simulink model "Fuzzy_pid_logic"  (R2025b)
settings: Solver=ode45  StartTime=0.0  StopTime=20  RelTol=1e-3
values from neighbouring files (symbols this model uses):
  ACE_norm = 0.20    (= 0.2)    [fuzzy_params.m]
  alpha = 0.002    [fuzzy_params.m]
  B = 0.425    [fuzzy_params.m]
  dACE_norm = 0.1    [fuzzy_params.m]
  Kd1 = Kp1 * Td1    (= 1.1799375)    [fuzzy_params.m]
  Kd2 = Kp2 * Td2    (= 0.2359875)    [fuzzy_params.m]
  Ki1 = Kp1 / Ti1    (= 0.00476720165263)    [fuzzy_params.m]
  Ki2 = Kp2 / Ti2    (= 0.000953440330526)    [fuzzy_params.m]
  Kp1 = 0.6 * Ku1    (= 0.15)    [fuzzy_params.m]
  Kp2 = 0.6 * Ku2    (= 0.03)    [fuzzy_params.m]
  Kps = 120    [fuzzy_params.m]
  Tg = 0.08    [fuzzy_params.m]
  TieGain = 2*pi*T12    (= 0.544123847602)    [fuzzy_params.m]
  Tps = 20    [fuzzy_params.m]
  Tt = 0.30    (= 0.3)    [fuzzy_params.m]
libraries: slpidlib x2, fuzblock x1
settings Model: Creator=parth  LastModifiedBy=parth
settings SolverCC: ZeroCrossAlgorithm=Adaptive
settings DebuggingCC: IgnoredZcDiagnostic=none

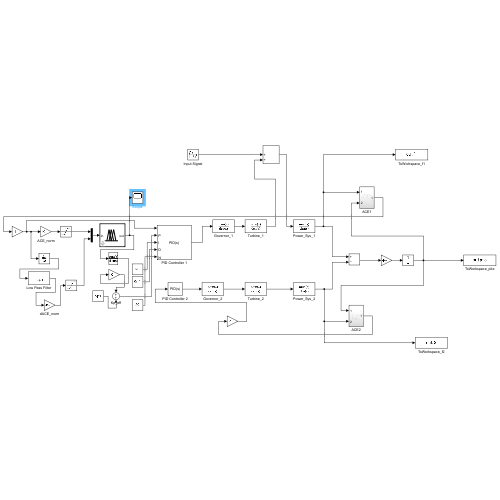
[thumbnail: Simulink's stored preview of the top-level diagram]
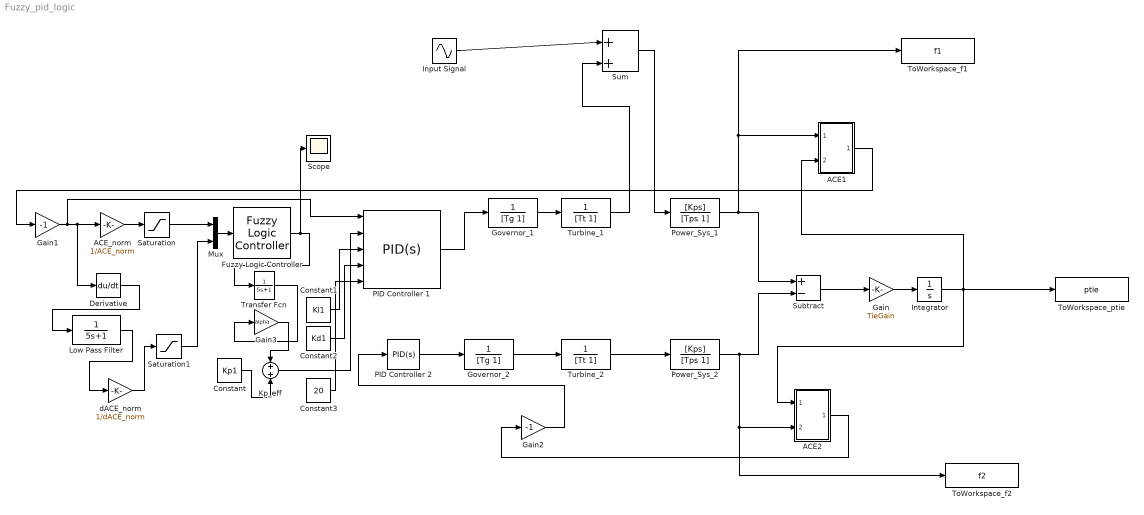
== system Fuzzy_pid_logic ==
  ACE1 : Subsystem
  ACE2 : Subsystem
  ACE_norm : Gain  Gain=1/ACE_norm
  Constant : Constant  Value=Kp1
  Constant1 : Constant  Value=Ki1
  Constant2 : Constant  Value=Kd1
  Constant3 : Constant  Value=20
  Derivative : Derivative  CoefficientInTFapproximation=1
  Fuzzy Logic Controller : fuzblock/Fuzzy Logic  Controller  FIS=fuzzy_pid  OutputSampleNumber=101  DataType=double  UseLookupTable=off  NumBreakpoints=10  FuzzifiedInputs=off  RuleFiringStrengths=off  RuleOutputs=off  AggregatedOutputs=off  SimulateUsing=Interpreted execution  OutOfRangeInputValueMessage=warning  NoRuleFiredMessage=warning  EmptyOutputFuzzySetMessage=warning
  Gain : Gain  Gain=TieGain
  Gain1 : Gain  Gain=-1
  Gain2 : Gain  Gain=-1
  Gain3 : Gain  Gain=alpha
  Governor_1 : TransferFcn  Denominator=[Tg 1]
  Governor_2 : TransferFcn  Denominator=[Tg 1]
  Input Signal : Sin  Amplitude=0.01  SampleTime=0
  Integrator : Integrator
  Kp_eff : Sum
  Low Pass Filter : TransferFcn  Denominator=[5 1]
  Mux : Mux  Inputs=2
  PID Controller 1 : slpidlib/PID Controller  Controller=PID  Form=Parallel  TimeDomain=Continuous-time  UseExternalTs=off  SampleTime=-1  IntegratorMethod=Forward Euler  FilterMethod=Forward Euler  ControllerParametersSource=external  P=Kp1  I=Ki1  UseKiTs=off  D=Kd1  UseExternalDerivativeSource=off  N=100  UseFilter=on  TunerSelectOption=Frequency Response Based  InitialConditionSource=internal  InitialConditionForIntegrator=0  InitialConditionForFilter=0  DifferentiatorICPrevScaledInput=0  ExternalReset=none  TrackingMode=off  Kt=1  LimitOutput=off  SatLimitsSource=internal  UpperSaturationLimit=inf  LowerSaturationLimit=-inf  LinearizeAsGain=on  AntiWindupMode=none  Kb=1  LimitIntegrator=off  UpperIntegratorSaturationLimit=inf  LowerIntegratorSaturationLimit=-inf  POutMin=[]  POutMax=[]  IOutMin=[]  IOutMax=[]  DOutMin=[]  DOutMax=[]  NOutMin=[]  NOutMax=[]  SumOutMin=[]  SumOutMax=[]  SaturationOutMin=[]  SaturationOutMax=[]  PParamMin=[]  PParamMax=[]  IParamMin=[]  IParamMax=[]  DParamMin=[]  DParamMax=[]  NParamMin=[]  NParamMax=[]  KbParamMin=[]  KbParamMax=[]  KtParamMin=[]  KtParamMax=[]  KbOutMin=[]  KbOutMax=[]  KtOutMin=[]  KtOutMax=[]  IntegratorOutMin=[]  IntegratorOutMax=[]  FilterOutMin=[]  FilterOutMax=[]  SumI1OutMin=[]  SumI1OutMax=[]  SumI2OutMin=[]  SumI2OutMax=[]  SumI3OutMin=[]  SumI3OutMax=[]  SumI4OutMin=[]  SumI4OutMax=[]  SumDOutMin=[]  SumDOutMax=[]  DifferentiatorOutMin=[]  DifferentiatorOutMax=[]  FilterDiffOutCoefMin=[]  FilterDiffOutCoefMax=[]  ReciprocalOutMin=[]  ReciprocalOutMax=[]  SumDenOutMin=[]  SumDenOutMax=[]  SumNumOutMin=[]  SumNumOutMax=[]  DivideOutMin=[]  DivideOutMax=[]  UdiffTsProdOutMin=[]  UdiffTsProdOutMax=[]  NTsProdOutMin=[]  NTsProdOutMax=[]  UintegralTsProdOutMin=[]  UintegralTsProdOutMax=[]  UngainTsProdOutMin=[]  UngainTsProdOutMax=[]  ClampingZeroOutDataTypeStr=Inherit: Inherit via back propagation  ClampingZeroOutMin=[]  ClampingZeroOutMax=[]  FilterDenConstantOutDataTypeStr=Inherit: Inherit via back propagation  FilterDenConstantOutMin=[]  FilterDenConstantOutMax=[]  PCopyOutDataTypeStr=Inherit: Inherit via back propagation  PCopyOutMin=[]  PCopyOutMax=[]  NCopyOutDataTypeStr=Inherit: Inherit via back propagation  NCopyOutMin=[]  NCopyOutMax=[]  IntegratorContinuousStateAttributes=''  IntegratorStateMustResolveToSignalObject=off  IntegratorRTWStateStorageClass=Auto  FilterContinuousStateAttributes=''  FilterStateMustResolveToSignalObject=off  FilterRTWStateStorageClass=Auto  ParallelPVariant=ExternalParameters  IdealPVariant=Disabled  IVariant=ExternalParameters  DVariant=ExternalParameters  IntegratorVariant=Continuous  SatVariant=Disabled  AWVariant=Passthrough  PCopyVariant=Disabled  TRVariant=Disabled  FdbkBlocksVariant=Forward  IdealPFdbkVariant=Disabled  SatFdbkVariant=Disabled  DerivativeFilterVariant=ContFilter  NVariant=ExternalParameters  NCopyVariant=Disabled  FilterICVariant=InternalICsFilter  IntegratorICVariant=InternalICs  ExternalResetVariant=Disabled  TRSumVariant=Passthrough  SumFdbkVariant=Disabled  SumVariant=Sum_PID  TsampFilterVariant=InternalTs  TsampNgainVariant=Passthrough  TsampIntegralVariant=Disabled_SignalSpec  ExternalSaturationOutDataTypeStr=Inherit: Same as second input  DerivativeSourceVariant=ErrorSignal  PreIntVariant=InternalPreInt
  PID Controller 2 : slpidlib/PID Controller  Controller=PID  Form=Parallel  TimeDomain=Continuous-time  UseExternalTs=off  SampleTime=-1  IntegratorMethod=Forward Euler  FilterMethod=Forward Euler  ControllerParametersSource=internal  P=Kp2  I=Ki2  UseKiTs=off  D=Kd2  UseExternalDerivativeSource=off  N=100  UseFilter=on  TunerSelectOption=Frequency Response Based  InitialConditionSource=internal  InitialConditionForIntegrator=0  InitialConditionForFilter=0  DifferentiatorICPrevScaledInput=0  ExternalReset=none  TrackingMode=off  Kt=1  LimitOutput=off  SatLimitsSource=internal  UpperSaturationLimit=inf  LowerSaturationLimit=-inf  LinearizeAsGain=on  AntiWindupMode=none  Kb=1  LimitIntegrator=off  UpperIntegratorSaturationLimit=inf  LowerIntegratorSaturationLimit=-inf  POutMin=[]  POutMax=[]  IOutMin=[]  IOutMax=[]  DOutMin=[]  DOutMax=[]  NOutMin=[]  NOutMax=[]  SumOutMin=[]  SumOutMax=[]  SaturationOutMin=[]  SaturationOutMax=[]  PParamMin=[]  PParamMax=[]  IParamMin=[]  IParamMax=[]  DParamMin=[]  DParamMax=[]  NParamMin=[]  NParamMax=[]  KbParamMin=[]  KbParamMax=[]  KtParamMin=[]  KtParamMax=[]  KbOutMin=[]  KbOutMax=[]  KtOutMin=[]  KtOutMax=[]  IntegratorOutMin=[]  IntegratorOutMax=[]  FilterOutMin=[]  FilterOutMax=[]  SumI1OutMin=[]  SumI1OutMax=[]  SumI2OutMin=[]  SumI2OutMax=[]  SumI3OutMin=[]  SumI3OutMax=[]  SumI4OutMin=[]  SumI4OutMax=[]  SumDOutMin=[]  SumDOutMax=[]  DifferentiatorOutMin=[]  DifferentiatorOutMax=[]  FilterDiffOutCoefMin=[]  FilterDiffOutCoefMax=[]  ReciprocalOutMin=[]  ReciprocalOutMax=[]  SumDenOutMin=[]  SumDenOutMax=[]  SumNumOutMin=[]  SumNumOutMax=[]  DivideOutMin=[]  DivideOutMax=[]  UdiffTsProdOutMin=[]  UdiffTsProdOutMax=[]  NTsProdOutMin=[]  NTsProdOutMax=[]  UintegralTsProdOutMin=[]  UintegralTsProdOutMax=[]  UngainTsProdOutMin=[]  UngainTsProdOutMax=[]  ClampingZeroOutDataTypeStr=Inherit: Inherit via back propagation  ClampingZeroOutMin=[]  ClampingZeroOutMax=[]  FilterDenConstantOutDataTypeStr=Inherit: Inherit via back propagation  FilterDenConstantOutMin=[]  FilterDenConstantOutMax=[]  PCopyOutDataTypeStr=Inherit: Inherit via back propagation  PCopyOutMin=[]  PCopyOutMax=[]  NCopyOutDataTypeStr=Inherit: Inherit via back propagation  NCopyOutMin=[]  NCopyOutMax=[]  IntegratorContinuousStateAttributes=''  IntegratorStateMustResolveToSignalObject=off  IntegratorRTWStateStorageClass=Auto  FilterContinuousStateAttributes=''  FilterStateMustResolveToSignalObject=off  FilterRTWStateStorageClass=Auto  ParallelPVariant=InternalParameters  IdealPVariant=Disabled  IVariant=InternalParameters  DVariant=InternalParameters  IntegratorVariant=Continuous  SatVariant=Disabled  AWVariant=Passthrough  PCopyVariant=Disabled  TRVariant=Disabled  FdbkBlocksVariant=Forward  IdealPFdbkVariant=Disabled  SatFdbkVariant=Disabled  DerivativeFilterVariant=ContFilter  NVariant=InternalParameters  NCopyVariant=Disabled  FilterICVariant=InternalICsFilter  IntegratorICVariant=InternalICs  ExternalResetVariant=Disabled  TRSumVariant=Passthrough  SumFdbkVariant=Disabled  SumVariant=Sum_PID  TsampFilterVariant=InternalTs  TsampNgainVariant=Passthrough  TsampIntegralVariant=Disabled_SignalSpec  ExternalSaturationOutDataTypeStr=Inherit: Same as second input  DerivativeSourceVariant=ErrorSignal  PreIntVariant=InternalPreInt
  Power_Sys_1 : TransferFcn  Numerator=[Kps]  Denominator=[Tps 1]
  Power_Sys_2 : TransferFcn  Numerator=[Kps]  Denominator=[Tps 1]
  Saturation : Saturate  UpperLimit=1  LowerLimit=-1  LinearizeAsGain=off  ZeroCross=off
  Saturation1 : Saturate  UpperLimit=1  LowerLimit=-1  LinearizeAsGain=off  ZeroCross=off
  Scope : Scope
      settings: ActiveDisplayYMinimum=-0.15656181660395219  ActiveDisplayYMaximum=0.10691571021676333
  Subtract : Sum  Inputs=+-
  Sum : Sum  Inputs=|++
  ToWorkspace_f1 : ToWorkspace  VariableName=f1  SampleTime=-1
      settings: Save2DSignal=2-D array (concatenate along first dimension)
  ToWorkspace_f2 : ToWorkspace  VariableName=f2  SampleTime=-1
      settings: Save2DSignal=2-D array (concatenate along first dimension)
  ToWorkspace_ptie : ToWorkspace  VariableName=ptie  SampleTime=-1
      settings: Save2DSignal=2-D array (concatenate along first dimension)
  Transfer Fcn : TransferFcn  Denominator=[5 1]
  Turbine_1 : TransferFcn  Denominator=[Tt 1]
  Turbine_2 : TransferFcn  Denominator=[Tt 1]
  dACE_norm : Gain  Gain=1/dACE_norm
  wires:
  Sum/1 -> Power_Sys_1/1
  Gain/1 -> Integrator/1
  Integrator/1 -> ACE1/2(In2), ToWorkspace_ptie/1, ACE2/1(In1)
  ACE1/1(Out1) -> Gain1/1
  Turbine_1/1 -> Sum/2
  Power_Sys_2/1 -> ToWorkspace_f2/1, ACE2/2(In2), Subtract/2
  ACE2/1(Out1) -> Gain2/1
  Subtract/1 -> Gain/1
  Governor_2/1 -> Turbine_2/1
  Governor_1/1 -> Turbine_1/1
  PID Controller 2/1 -> Governor_2/1
  Gain2/1 -> PID Controller 2/1
  Power_Sys_1/1 -> ToWorkspace_f1/1, ACE1/1(In1), Subtract/1
  Turbine_2/1 -> Power_Sys_2/1
  Input Signal/1 -> Sum/1
  Gain1/1 -> PID Controller 1/1, Derivative/1, ACE_norm/1
  Mux/1 -> Fuzzy Logic Controller/1
  ACE_norm/1 -> Saturation/1
  Saturation/1 -> Mux/1
  Saturation1/1 -> Mux/2
  dACE_norm/1 -> Saturation1/1
  Derivative/1 -> Low Pass Filter/1
  Low Pass Filter/1 -> dACE_norm/1
  Fuzzy Logic Controller/1 -> Scope/1, Transfer Fcn/1
  Transfer Fcn/1 -> Gain3/1
  Constant/1 -> Kp_eff/2
  Kp_eff/1 -> PID Controller 1/2
  Constant1/1 -> PID Controller 1/3
  Constant2/1 -> PID Controller 1/4
  Constant3/1 -> PID Controller 1/5
  PID Controller 1/1 -> Governor_1/1
  Gain3/1 -> Kp_eff/1

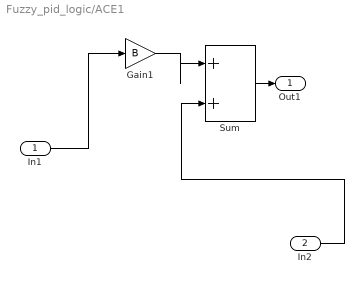
== system Fuzzy_pid_logic/ACE1 ==
  In1 : Inport
  In2 : Inport  Port=2
  Gain1 : Gain  Gain=B
  Sum : Sum  Inputs=|++
  Out1 : Outport
  wires:
  In1/1 -> Gain1/1
  Gain1/1 -> Sum/1
  Sum/1 -> Out1/1
  In2/1 -> Sum/2

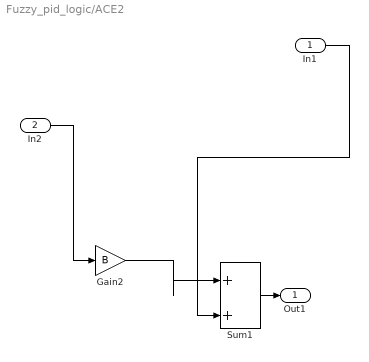
== system Fuzzy_pid_logic/ACE2 ==
  In1 : Inport
  In2 : Inport  Port=2
  Gain2 : Gain  Gain=B
  Sum1 : Sum  Inputs=|++
  Out1 : Outport
  wires:
  Gain2/1 -> Sum1/1
  In2/1 -> Gain2/1
  In1/1 -> Sum1/2
  Sum1/1 -> Out1/1
